simulink model "ABSBang"  (R2020a)
settings: Solver=VariableStepAuto  StartTime=0.0  StopTime=90  RelTol=1e-3
values from neighbouring files (symbols this model uses):
  A = 48.87    [ABSData.m]
  g = 9.806    [ABSData.m]    (also in ABScode.m)
  J = 4.077    [ABSData.m]    (also in ABScode.m)
  m = 26    [ABSData.m]    (also in ABScode.m = 255)
  mu = 0.52    [ABSData.m]
  P = 1.9    [ABSData.m]
  r = 0.32    [ABSData.m]
  R = 0.636    [ABSData.m]    (also in ABScode.m = 1.635)
  v0 = 50    [ABSData.m]    (also in ABScode.m = 80)
settings Model: Creator=Stephen Kingston  LastModifiedBy=Ghani
settings SFSimCC: CustomCodeUndefinedFunction=UseInterfaceOnly

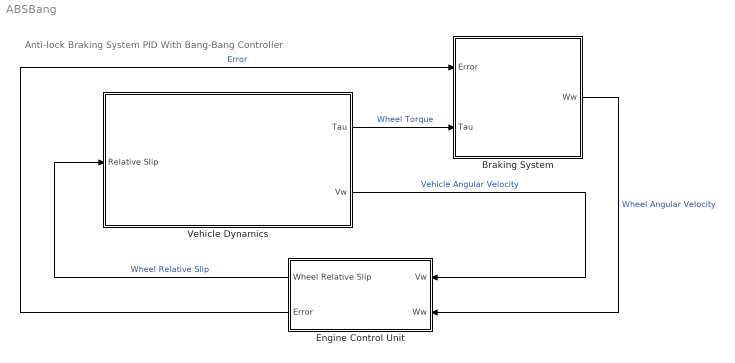
== system ABSBang ==
  note: Anti-lock Braking System PID With Bang-Bang Controller
  Braking System : Subsystem
      mask Display: image('Front.jpg'); % Use "Edit Image" on toolstrip to change.
  Engine Control Unit : Subsystem
      mask Display: image('ECU.png'); % Use "Edit Image" on toolstrip to change.
  Vehicle Dynamics : Subsystem
      mask Display: image('Full System.jpg'); % Use "Edit Image" on toolstrip to change.
  wires:
  Engine Control Unit/1(Wheel Relative Slip) -> Vehicle Dynamics/1(Relative Slip)  "Wheel Relative Slip"
  Vehicle Dynamics/1(Tau) -> Braking System/2(Tau)  "Wheel Torque"
  Vehicle Dynamics/2(Vw) -> Engine Control Unit/1(Vw)  "Vehicle Angular Velocity"
  Braking System/1(Ww) -> Engine Control Unit/2(Ww)  "Wheel Angular Velocity"
  Engine Control Unit/2(Error) -> Braking System/1(Error)  "Error"

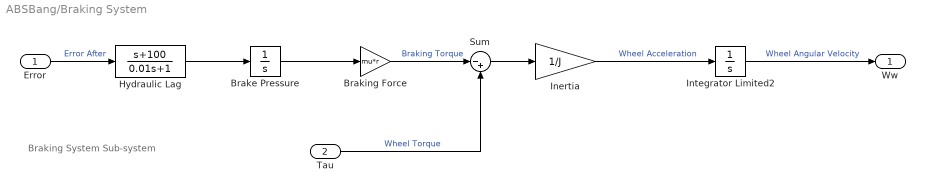
== system ABSBang/Braking System ==
  note: Braking System Sub-system
  Error : Inport
  Tau : Inport  Port=2
  Brake Pressure : Integrator  InitialCondition=P*A  LimitOutput=on  UpperSaturationLimit=1500  LowerSaturationLimit=0
  Braking Force : Gain  Gain=mu*r
  Hydraulic Lag : TransferFcn  Numerator=[1 100]  Denominator=[0.01 1]
  Inertia : Gain  Gain=1/J
  Integrator Limited2 : Integrator  InitialCondition=v0/R  LimitOutput=on  UpperSaturationLimit=1000  LowerSaturationLimit=0
  Sum : Sum  Inputs=|-+
  Ww : Outport  VectorParamsAs1DForOutWhenUnconnected=off
  wires:
  Inertia/1 -> Integrator Limited2/1  "Wheel Acceleration"
  Integrator Limited2/1 -> Ww/1  "Wheel Angular Velocity"
  Tau/1 -> Sum/2  "Wheel Torque"
  Hydraulic Lag/1 -> Brake Pressure/1
  Sum/1 -> Inertia/1
  Error/1 -> Hydraulic Lag/1  "Error After"
  Braking Force/1 -> Sum/1  "Braking Torque"
  Brake Pressure/1 -> Braking Force/1

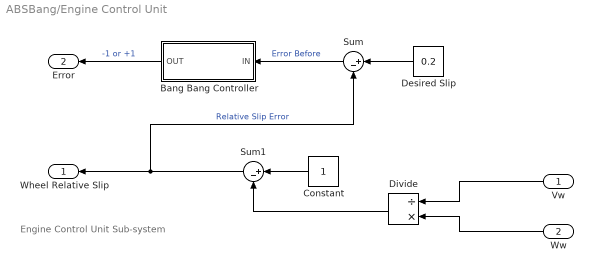
== system ABSBang/Engine Control Unit ==
  note: Engine Control Unit Sub-system
  Vw : Inport
  Ww : Inport  Port=2
  Bang Bang Controller : Subsystem
      mask Display: image('C:\Users\Ghani\Downloads\moto - Copy.png'); % Use "Edit Image" on toolstrip to change.
  Constant : Constant
  "Desired Slip " : Constant  Value=0.2
  Divide : Product  Inputs=/*
  Sum : Sum  Inputs=|+-
  Sum1 : Sum  Inputs=|+-
  Wheel Relative Slip : Outport  VectorParamsAs1DForOutWhenUnconnected=off
  Error : Outport  Port=2
  wires:
  Constant/1 -> Sum1/1
  Ww/1 -> Divide/2
  Vw/1 -> Divide/1
  Divide/1 -> Sum1/2
  Sum1/1 -> Wheel Relative Slip/1, Sum/2  "Relative Slip Error"
  Sum/1 -> Bang Bang Controller/1(IN)  "Error Before"
  Bang Bang Controller/1(OUT) -> Error/1  "-1 or +1"
  "Desired Slip "/1 -> Sum/1

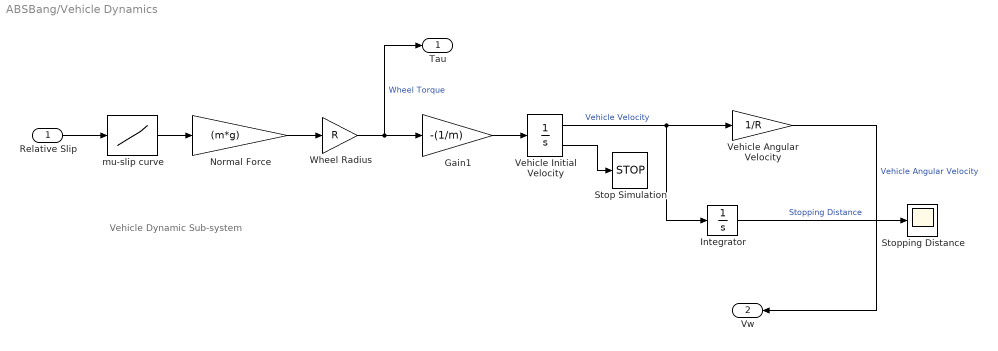
== system ABSBang/Vehicle Dynamics ==
  note: Vehicle Dynamic Sub-system
  Relative Slip : Inport
  Gain1 : Gain  Gain=-(1/m)
  Integrator : Integrator
  Normal Force : Gain  Gain=(m*g)
  Stop Simulation : Stop
  Stopping Distance : Scope
  Vehicle Angular Velocity : Gain  Gain=1/R
  Vehicle Initial Velocity : Integrator  InitialCondition=v0  LimitOutput=on  UpperSaturationLimit=1000  LowerSaturationLimit=0  ShowSaturationPort=on
  Wheel Radius : Gain  Gain=R
  mu-slip curve : Lookup_n-D  NumberOfTableDimensions=1  BreakpointsForDimension1=[0,0.025,0.05,0.075,0.1,0.125,0.15,0.175,0.2,0.225,0.25,0.275,0.3,0.325,0.35,0.375,0.4,0.425,0.45,0.475,0.5,0.525,0.55,0.575,0.6,0.625,0.65,0.675,0.7,0.725,0.75,0.775,0.8,0.825,0.85,0.875,0.9,0.925,0.95,0.975,1]  Table=[0,0.3,0.75,1,1.15,1.16,1.17,1.18,1.17,1.16,1.15,1.14,1.125,1.1,1.09,1.075,1.06,1.045,1.03,1.015,1,0.99,0.98,0.97,0.96,0.95,0.94,0.93,0.92,0.91,0.9,0.89,0.88,0.87,0.86,0.85,0.835,0.82,0.81,0.80,0.79]  RndMeth=Simplest  InputSameDT=on
  Tau : Outport
  Vw : Outport  Port=2
  wires:
  Vehicle Initial Velocity/2 -> Stop Simulation/1
  Vehicle Initial Velocity/1 -> Vehicle Angular Velocity/1, Integrator/1  "Vehicle Velocity"
  Normal Force/1 -> Wheel Radius/1
  Gain1/1 -> Vehicle Initial Velocity/1
  Wheel Radius/1 -> Tau/1, Gain1/1  "Wheel Torque"
  mu-slip curve/1 -> Normal Force/1
  Relative Slip/1 -> mu-slip curve/1
  Integrator/1 -> Stopping Distance/1  "Stopping Distance"
  Vehicle Angular Velocity/1 -> Vw/1  "Vehicle Angular Velocity"

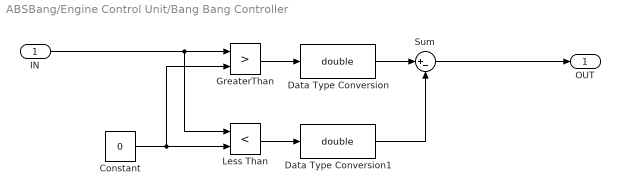
== system ABSBang/Engine Control Unit/Bang Bang Controller ==
  IN : Inport
  Constant : Constant  Value=0
  Data Type Conversion : DataTypeConversion  OutDataTypeStr=double  RndMeth=Zero
  Data Type Conversion1 : DataTypeConversion  OutDataTypeStr=double  RndMeth=Zero
  GreaterThan : RelationalOperator  Operator=>  OutDataTypeStr=boolean  RndMeth=Simplest
  Less Than : RelationalOperator  Operator=<  OutDataTypeStr=boolean  RndMeth=Simplest
  Sum : Sum  Inputs=|+-
  OUT : Outport  VectorParamsAs1DForOutWhenUnconnected=off
  wires:
  Sum/1 -> OUT/1
  Data Type Conversion/1 -> Sum/1
  Constant/1 -> Less Than/2, GreaterThan/2
  IN/1 -> Less Than/1, GreaterThan/1
  Data Type Conversion1/1 -> Sum/2
  GreaterThan/1 -> Data Type Conversion/1
  Less Than/1 -> Data Type Conversion1/1
